simulink model "skyhook_suspension"  (R2025a)
settings: Solver=ode23s  StartTime=0.0  StopTime=T_sim  RelTol=1e-3
undefined symbols (not defined in the file): cs_off, cs_on, ks, kt, ms, mus, zs_static, zus_static
settings Model: Creator=Anderson  LastModifiedBy=Anderson
settings DataIOCC: SaveFormat=Array

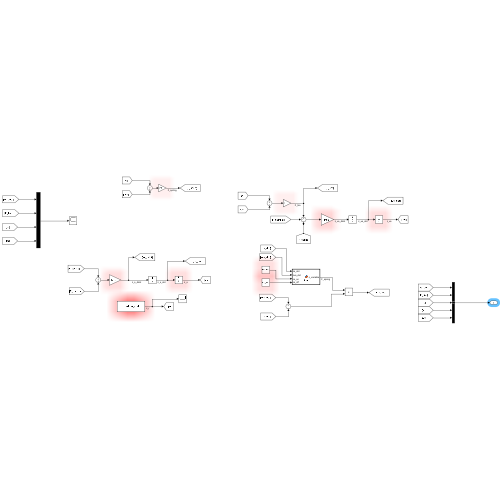
[thumbnail: Simulink's stored preview of the top-level diagram]
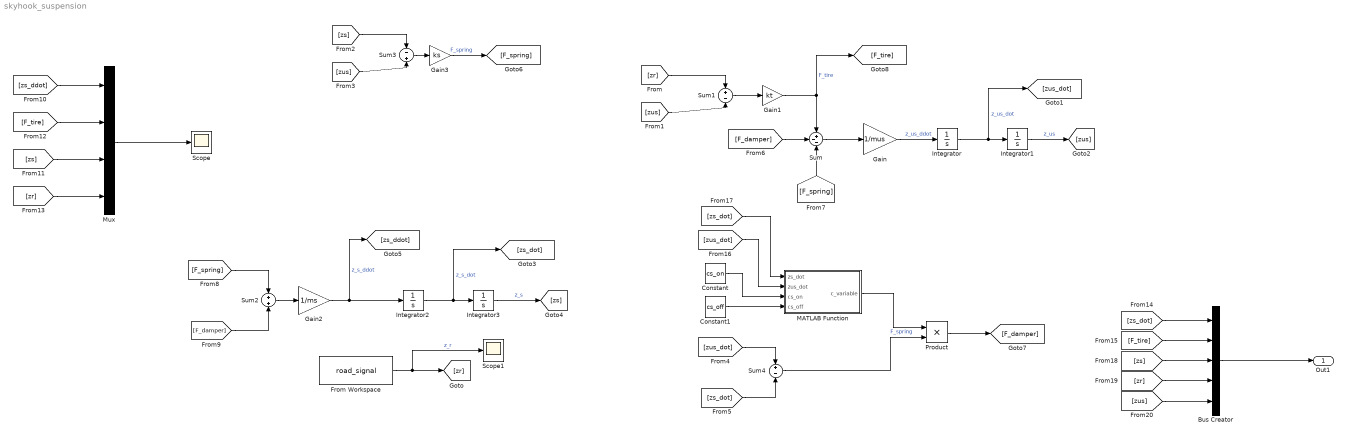
== system skyhook_suspension ==
  Bus Creator : BusCreator  Inputs=5
  Constant : Constant  Value=cs_on
  Constant1 : Constant  Value=cs_off
  From Workspace : FromWorkspace  VariableName=road_signal
  Gain : Gain  Gain=1/mus
  Gain1 : Gain  Gain=kt
  Gain2 : Gain  Gain=1/ms
  Gain3 : Gain  Gain=ks
  Integrator : Integrator
  Integrator1 : Integrator  InitialCondition=zus_static
  Integrator2 : Integrator
  Integrator3 : Integrator  InitialCondition=zs_static
  MATLAB Function : MATLAB Function  TreatAsAtomicUnit=on
  Mux : Mux
  Product : Product
  Scope : Scope
      settings: ActiveDisplayYMinimum=-6868.1819363859859  ActiveDisplayYMaximum=4567.23132626511
  Scope1 : Scope
      settings: ActiveDisplayYMinimum=-0.012493378905301503  ActiveDisplayYMaximum=0.11244041014771355
  Sum : Sum  Inputs=+--
  Sum1 : Sum  Inputs=+-
  Sum2 : Sum
  Sum3 : Sum  Inputs=-+
  Sum4 : Sum  Inputs=+-
  Out1 : Outport
  wires:
  From Workspace/1 -> [zr], Scope1/1  "z_r"
  Integrator/1 -> [zus_dot], Integrator1/1  "z_us_dot"
  Gain/1 -> Integrator/1  "z_us_ddot​"
  Integrator1/1 -> [zus]  "z_us"
  Sum/1 -> Gain/1
  [zr] -> Sum1/1
  [zus] -> Sum1/2
  Sum1/1 -> Gain1/1
  Gain1/1 -> Sum/1, [F_tire]  "F_tire"
  Gain2/1 -> [zs_ddot], Integrator2/1  "z_s_ddot"
  Integrator2/1 -> [zs_dot], Integrator3/1  "z_s_dot"
  Integrator3/1 -> [zs]  "z_s"
  Sum2/1 -> Gain2/1
  [zs] -> Sum3/1
  [zus] -> Sum3/2
  Sum3/1 -> Gain3/1
  Gain3/1 -> [F_spring]  "F_spring"
  [zus_dot] -> Sum4/1
  [zs_dot] -> Sum4/2
  Sum4/1 -> Product/2
  Product/1 -> [F_damper]
  [F_spring] -> Sum/3
  [F_damper] -> Sum/2
  [F_spring] -> Sum2/1
  [F_damper] -> Sum2/2
  [zs_ddot] -> Mux/1
  [F_tire] -> Mux/2
  [zs] -> Mux/3
  [zr] -> Mux/4
  Mux/1 -> Scope/1
  [zs_dot] -> MATLAB Function/1(zs_dot)
  [zus_dot] -> MATLAB Function/2(zus_dot)
  MATLAB Function/1(c_variable) -> Product/1  "F_spring"
  Constant/1 -> MATLAB Function/3(cs_on)
  Constant1/1 -> MATLAB Function/4(cs_off)
  [zus] -> Bus Creator/5
  [zr] -> Bus Creator/4
  [zs] -> Bus Creator/3
  [F_tire] -> Bus Creator/2
  [zs_dot] -> Bus Creator/1
  Bus Creator/1 -> Out1/1

== matlab function skyhook_suspension/MATLAB Function ==
  data: zs_dot input; c_variable output; zus_dot input; cs_on input; cs_off input
function c_variable = fcn(zs_dot, zus_dot, cs_on, cs_off)
%#codegen

% Esta função implementa a lógica de controle Skyhook On-Off.
% As variáveis cs_on e cs_off são lidas do base workspace.

if zs_dot * (zs_dot - zus_dot) >= 0
    % Condição "céu": amortecedor atua para frear o chassi
    c_variable = cs_on;
else
    % Condição "chão": amortecedor fica "mole" para não atrapalhar
    c_variable = cs_off;
end
